simulink model "subsystem_calculator"  (R2017b)
settings: Solver=FixedStepDiscrete  StartTime=0.0  StopTime=10.0  RelTol=1e-3
settings Model: Creator=ibrahim  LastModifiedBy=ibrahim
settings OptimizationCC: DefaultParameterBehavior=Inlined  PassReuseOutputArgsAs=Individual arguments
settings DebuggingCC: ParameterTunabilityLossMsg=error
settings SFSimCC: MATLABDynamicMemAlloc=off
settings RTWCC: SystemTargetFile=ert.tlc  GenCodeOnly=on  TemplateMakefile=ert_default_tmf  GenerateReport=on  IncludeHyperlinkInReport=on  LaunchReport=on  GenerateTraceInfo=on  GenerateTraceReport=on  GenerateTraceReportSl=on  GenerateTraceReportSf=on  GenerateTraceReportEml=on  GenerateWebview=on
settings CodeAppCC: ForceParamTrailComments=on  IgnoreCustomStorageClasses=off  OperatorAnnotations=on  SimulinkDataObjDesc=on  SFDataObjDesc=on  InsertBlockDesc=on
settings ERTTargetCC: TargetLangStandard=C99 (ISO)  GenerateSampleERTMain=on  InlinedParameterPlacement=NonHierarchical  ERTCustomFileTemplate=example_file_process.tlc

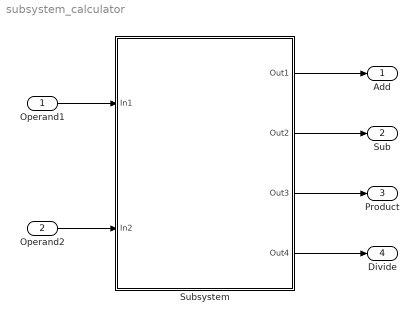
== system subsystem_calculator ==
  Operand1 : Inport
  Operand2 : Inport  Port=2
  Subsystem : Subsystem
  Add : Outport
  Sub : Outport  Port=2
  Product : Outport  Port=3
  Divide : Outport  Port=4
  wires:
  Operand1/1 -> Subsystem/1(In1)
  Operand2/1 -> Subsystem/2(In2)
  Subsystem/1(Out1) -> Add/1
  Subsystem/2(Out2) -> Sub/1
  Subsystem/3(Out3) -> Product/1
  Subsystem/4(Out4) -> Divide/1

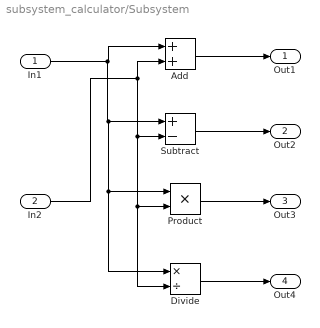
== system subsystem_calculator/Subsystem ==
  In1 : Inport
  In2 : Inport  Port=2
  Add : Sum
  Divide : Product  Inputs=*/
  Product : Product
  Subtract : Sum  Inputs=+-
  Out1 : Outport
  Out2 : Outport  Port=2
  Out3 : Outport  Port=3
  Out4 : Outport  Port=4
  wires:
  In1/1 -> Divide/1, Product/1, Subtract/1, Add/1
  In2/1 -> Divide/2, Product/2, Subtract/2, Add/2
  Add/1 -> Out1/1
  Subtract/1 -> Out2/1
  Product/1 -> Out3/1
  Divide/1 -> Out4/1
